simulink model "Ques2_system"  (R2020b)
settings: Solver=VariableStepAuto  StartTime=0.0  StopTime=100  RelTol=1e-3
settings Model: Creator=sneha  LastModifiedBy=sneha
settings DataIOCC: ExternalInput=[t, road_signal]  LoadExternalInput=on  SaveFormat=Array

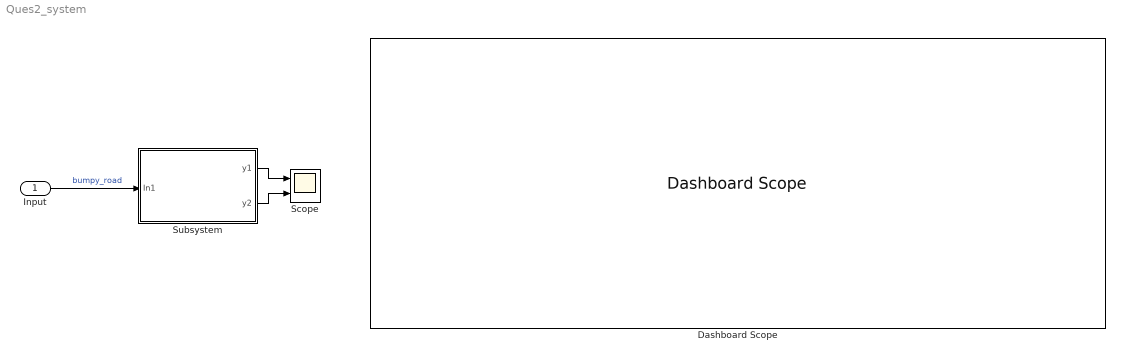
== system Ques2_system ==
  Input : Inport
  Dashboard Scope : DashboardScope
  Scope : Scope  NumInputPorts=2
  Subsystem : Subsystem  mask{m1=0, m2=0, k1=0, k2=0, b=0}
      mask prompts: m1 "mass1"; m2 "mass2"; k1 "spring constant 1"; k2 "spring constant 2"; b "damper"
  wires:
  Input/1 -> Subsystem/1(In1)  "bumpy_road"
  Subsystem/1(y1) -> Scope/1
  Subsystem/2(y2) -> Scope/2

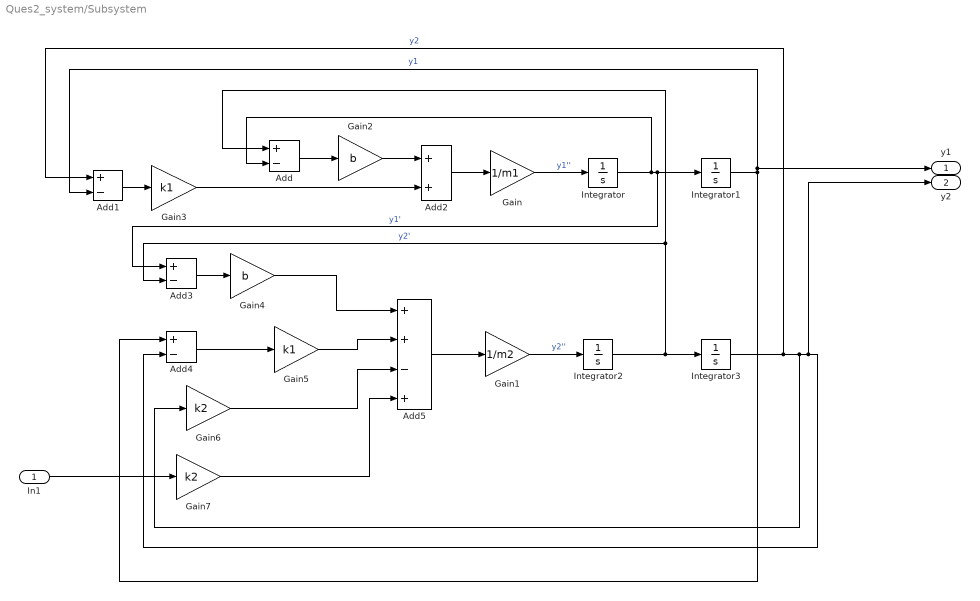
== system Ques2_system/Subsystem ==
  In1 : Inport
  Add{,1,3..4} (4 alike) : Sum  Inputs=+-
  Add2 : Sum
  Add5 : Sum  Inputs=++-+
  Gain : Gain  Gain=1/m1
  Gain1 : Gain  Gain=1/m2
  Gain2 : Gain  Gain=b
  Gain3 : Gain  Gain=k1
  Gain4 : Gain  Gain=b
  Gain5 : Gain  Gain=k1
  Gain6 : Gain  Gain=k2
  Gain7 : Gain  Gain=k2
  Integrator{,1..3} (4 alike) : Integrator
  y1 : Outport
  y2 : Outport  Port=2
  wires:
  Gain3/1 -> Add2/2
  Integrator1/1 -> y1/1, Add1/2, Add4/1  "y1"
  Gain1/1 -> Integrator2/1  "y2''"
  Gain/1 -> Integrator/1  "y1''"
  Integrator/1 -> Add3/1, Integrator1/1, Add/2  "y1'"
  Integrator2/1 -> Add3/2, Add/1, Integrator3/1  "y2'"
  Add1/1 -> Gain3/1
  Gain5/1 -> Add5/2
  Gain6/1 -> Add5/3
  Add4/1 -> Gain5/1
  Integrator3/1 -> Gain6/1, y2/1, Add4/2, Add1/1  "y2"
  Add3/1 -> Gain4/1
  Gain7/1 -> Add5/4
  Gain2/1 -> Add2/1
  Add2/1 -> Gain/1
  Add/1 -> Gain2/1
  Gain4/1 -> Add5/1
  Add5/1 -> Gain1/1
  In1/1 -> Gain7/1
